simulink model "five_tank_hybrid_system"  (R2019a)
settings: Solver=FixedStepDiscrete  StartTime=0.0  StopTime=T  FixedStep=Ts  RelTol=1e-3
InitFcn:
  | load_parameters
values from neighbouring files (symbols this model uses):
  A1u = 0.0573+0.00286    (= 0.06016)    [load_parameters.m]
  A2u = 0.0573+0.00286    (= 0.06016)    [load_parameters.m]
  A3u = 0.0346+0.0017    (= 0.0363)    [load_parameters.m]
  A4u = 0.0346+0.0017    (= 0.0363)    [load_parameters.m]
  A5u = 0.0707+0.00353    (= 0.07423)    [load_parameters.m]
  Ap1u = 3.167e-5+6.33e-6    (= 3.8e-05)    [load_parameters.m]
  Ap2u = 3.167e-5+6.33e-6    (= 3.8e-05)    [load_parameters.m]
  Ap3u = 3.167e-5+6.33e-6    (= 3.8e-05)    [load_parameters.m]
  Ap4u = 3.167e-5+6.33e-6    (= 3.8e-05)    [load_parameters.m]
  Ap5u = 3.167e-5+6.33e-6    (= 3.8e-05)    [load_parameters.m]
  Av1u = 3.167e-5+6.33e-6    (= 3.8e-05)    [load_parameters.m]
  Av2u = 3.167e-5+6.33e-6    (= 3.8e-05)    [load_parameters.m]
  Av3u = 3.167e-5+6.33e-6    (= 3.8e-05)    [load_parameters.m]
  Av4u = 3.167e-5+6.33e-6    (= 3.8e-05)    [load_parameters.m]
  cp1u = 0.68-0.0675    (= 0.6125)    [load_parameters.m]
  cp2u = 0.68-0.0675    (= 0.6125)    [load_parameters.m]
  cp3u = 0.4-0.038    (= 0.362)    [load_parameters.m]
  cp4u = 0.4-0.038    (= 0.362)    [load_parameters.m]
  cp5u = 0.7-0.068    (= 0.632)    [load_parameters.m]
  cv1u = 0.62-0.0615    (= 0.5585)    [load_parameters.m]
  cv2u = 0.62-0.0615    (= 0.5585)    [load_parameters.m]
  cv3u = 0.37-0.0365    (= 0.3335)    [load_parameters.m]
  cv4u = 0.37-0.0365    (= 0.3335)    [load_parameters.m]
  g = 9.81    [load_parameters.m]
  rho1 = 0.005    [load_parameters.m]
  rho2 = 0.005    [load_parameters.m]
  rho3 = 0.005    [load_parameters.m]
  rho4 = 0.005    [load_parameters.m]
  rho5 = 0.0063    [load_parameters.m]
  Ts = 0.01    [load_parameters.m]
  v = 0.02    [load_parameters.m]
  x1_0 = 0.3    [load_parameters.m]
  X1max = 0.4    [load_parameters.m]
  X1min = 0.1    [load_parameters.m]
  X1overflow = 0.405    [load_parameters.m]
  x2_0 = 0.12    [load_parameters.m]
  X2max = 0.4    [load_parameters.m]
  X2min = 0.1    [load_parameters.m]
  X2overflow = 0.405    [load_parameters.m]
  x3_0 = 0.15    [load_parameters.m]
  X3max = 0.35    [load_parameters.m]
  X3min = 0.1    [load_parameters.m]
  X3overflow = 0.355    [load_parameters.m]
  x4_0 = 0.3    [load_parameters.m]
  X4max = 0.35    [load_parameters.m]
  X4min = 0.1    [load_parameters.m]
  X4overflow = 0.355    [load_parameters.m]
  x5_0 = 0.09    [load_parameters.m]
  X5max = 0.2    [load_parameters.m]
  X5min = 0.05    [load_parameters.m]
  X5overflow = 0.205    [load_parameters.m]
  xi = 0.02    [load_parameters.m]
undefined symbols (not defined in the file or in its folder): dfilt, DiscIntNeverNeededParam
libraries: dsparch4 x5
(part 2 of 2)

== stateflow chart five_tank_hybrid_system/A9_Valve1/Chart ==
  state Stuck_Open
    entry: q=4;
  state Close
    entry: q=1;
  state Open
    entry: q=2;
  state Stuck_Close
    entry: q=3;
  Close -> Stuck_Open [order 2] : [phi10==1]
  Open -> Stuck_Open [order 2] : [phi10==1]
  (default) -> Close
  Close -> Open [order 1] : [x3<=X3min]
  Open -> Close [order 1] : [x3>=X3max]
  Close -> Stuck_Close [order 3] : [phi9==1]
  Open -> Stuck_Close [order 3] : [phi9==1]
  data: x3 input; phi9 input; phi10 input; X3min parameter; X3max parameter; q output

== matlab function five_tank_hybrid_system/A9_Valve1/MATLAB Function ==
  data: cv input; z output; Av input; in1 input; g input
function z = fm(cv,Av,in1,g)

z = cv*Av*sqrt(2*g*in1);

== stateflow chart five_tank_hybrid_system/A10_Valve2/Chart ==
  state Stuck_Open
    entry: q=4;
  state Close
    entry: q=1;
  state Open
    entry: q=2;
  state Stuck_Close
    entry: q=3;
  Close -> Stuck_Open [order 2] : [phi12==1]
  Open -> Stuck_Open [order 2] : [phi12==1]
  (default) -> Close
  Close -> Open [order 1] : [x4<=X4min]
  Open -> Close [order 1] : [x4>=X4max]
  Close -> Stuck_Close [order 3] : [phi11==1]
  Open -> Stuck_Close [order 3] : [phi11==1]
  data: x4 input; X4max parameter; X4min parameter; phi11 input; phi12 input; q output

== matlab function five_tank_hybrid_system/A10_Valve2/MATLAB Function ==
  data: cv input; z output; Av input; in1 input; g input
function z = fm(cv,Av,in1,g)

z = cv*Av*sqrt(2*g*in1);

== stateflow chart five_tank_hybrid_system/Scenarios/Healhy Scenario/Healthy ==
  state Healthy
    entry: phi1=0;
    entry: phi2=0;
    entry: phi3=0;
    entry: phi4=0;
    entry: phi5=0;
    entry: phi6=0;
    entry: phi7=0;
    entry: phi8=0;
    entry: phi9=0;
    entry: phi10=0;
    entry: phi11=0;
    entry: phi12=0;
    entry: phi13=0;
    entry: phi14=0;
    entry: phi15=0;
    entry: phi16=0;
  (default) -> Healthy
  data: phi1 output; phi2 output; phi3 output; phi4 output; phi5 output; phi6 output; phi7 output; phi8 output; phi9 output; phi10 output; phi11 output; phi12 output; phi13 output; phi14 output; phi15 output; phi16 output

== stateflow chart five_tank_hybrid_system/Scenarios/Leak Tank 1/Leak Tank 1 ==
  state Healthy
    entry: phi1=0;
    entry: phi2=0;
    entry: phi3=0;
    entry: phi4=0;
    entry: phi5=0;
    entry: phi6=0;
    entry: phi7=0;
    entry: phi8=0;
    entry: phi9=0;
    entry: phi10=0;
    entry: phi11=0;
    entry: phi12=0;
    entry: phi13=0;
    entry: phi14=0;
    entry: phi15=0;
    entry: phi16=0;
  state Fault
    entry: phi1=1;
    entry: phi2=0;
    entry: phi3=0;
    entry: phi4=0;
    entry: phi5=0;
    entry: phi6=0;
    entry: phi7=0;
    entry: phi8=0;
    entry: phi9=0;
    entry: phi10=0;
    entry: phi11=0;
    entry: phi12=0;
    entry: phi13=0;
    entry: phi14=0;
    entry: phi15=0;
    entry: phi16=0;
  (default) -> Healthy
  Healthy -> Fault : [t>Tf]
  data: phi1 output; phi2 output; phi3 output; phi4 output; phi5 output; phi6 output; phi7 output; phi8 output; phi9 output; phi10 output; phi11 output; phi12 output; phi13 output; phi14 output; phi15 output; phi16 output; Tf input

== stateflow chart five_tank_hybrid_system/Scenarios/Leak Tank 2/Leak Tank 2 ==
  state Healthy
    entry: phi1=0;
    entry: phi2=0;
    entry: phi3=0;
    entry: phi4=0;
    entry: phi5=0;
    entry: phi6=0;
    entry: phi7=0;
    entry: phi8=0;
    entry: phi9=0;
    entry: phi10=0;
    entry: phi11=0;
    entry: phi12=0;
    entry: phi13=0;
    entry: phi14=0;
    entry: phi15=0;
    entry: phi16=0;
  state Fault
    entry: phi1=0;
    entry: phi2=1;
    entry: phi3=0;
    entry: phi4=0;
    entry: phi5=0;
    entry: phi6=0;
    entry: phi7=0;
    entry: phi8=0;
    entry: phi9=0;
    entry: phi10=0;
    entry: phi11=0;
    entry: phi12=0;
    entry: phi13=0;
    entry: phi14=0;
    entry: phi15=0;
    entry: phi16=0;
  (default) -> Healthy
  Healthy -> Fault : [t>Tf]
  data: phi1 output; phi2 output; phi3 output; phi4 output; phi5 output; phi6 output; phi7 output; phi8 output; phi9 output; phi10 output; phi11 output; phi12 output; phi13 output; phi14 output; phi15 output; phi16 output; Tf input

== stateflow chart five_tank_hybrid_system/Scenarios/Leak Tank 3/Leak Tank 2 ==
  state Healthy
    entry: phi1=0;
    entry: phi2=0;
    entry: phi3=0;
    entry: phi4=0;
    entry: phi5=0;
    entry: phi6=0;
    entry: phi7=0;
    entry: phi8=0;
    entry: phi9=0;
    entry: phi10=0;
    entry: phi11=0;
    entry: phi12=0;
    entry: phi13=0;
    entry: phi14=0;
    entry: phi15=0;
    entry: phi16=0;
  state Fault
    entry: phi1=0;
    entry: phi2=0;
    entry: phi3=1;
    entry: phi4=0;
    entry: phi5=0;
    entry: phi6=0;
    entry: phi7=0;
    entry: phi8=0;
    entry: phi9=0;
    entry: phi10=0;
    entry: phi11=0;
    entry: phi12=0;
    entry: phi13=0;
    entry: phi14=0;
    entry: phi15=0;
    entry: phi16=0;
  (default) -> Healthy
  Healthy -> Fault : [t>Tf]
  data: phi1 output; phi2 output; phi3 output; phi4 output; phi5 output; phi6 output; phi7 output; phi8 output; phi9 output; phi10 output; phi11 output; phi12 output; phi13 output; phi14 output; phi15 output; phi16 output; Tf input

== stateflow chart five_tank_hybrid_system/Scenarios/Leak Tank 4/Leak Tank 4 ==
  state Healthy
    entry: phi1=0;
    entry: phi2=0;
    entry: phi3=0;
    entry: phi4=0;
    entry: phi5=0;
    entry: phi6=0;
    entry: phi7=0;
    entry: phi8=0;
    entry: phi9=0;
    entry: phi10=0;
    entry: phi11=0;
    entry: phi12=0;
    entry: phi13=0;
    entry: phi14=0;
    entry: phi15=0;
    entry: phi16=0;
  state Fault
    entry: phi1=0;
    entry: phi2=0;
    entry: phi3=0;
    entry: phi4=1;
    entry: phi5=0;
    entry: phi6=0;
    entry: phi7=0;
    entry: phi8=0;
    entry: phi9=0;
    entry: phi10=0;
    entry: phi11=0;
    entry: phi12=0;
    entry: phi13=0;
    entry: phi14=0;
    entry: phi15=0;
    entry: phi16=0;
  (default) -> Healthy
  Healthy -> Fault : [t>Tf]
  data: phi1 output; phi2 output; phi3 output; phi4 output; phi5 output; phi6 output; phi7 output; phi8 output; phi9 output; phi10 output; phi11 output; phi12 output; phi13 output; phi14 output; phi15 output; phi16 output; Tf input

== stateflow chart five_tank_hybrid_system/Scenarios/Leak Tank 5/Leak Tank 5 ==
  state Healthy
    entry: phi1=0;
    entry: phi2=0;
    entry: phi3=0;
    entry: phi4=0;
    entry: phi5=0;
    entry: phi6=0;
    entry: phi7=0;
    entry: phi8=0;
    entry: phi9=0;
    entry: phi10=0;
    entry: phi11=0;
    entry: phi12=0;
    entry: phi13=0;
    entry: phi14=0;
    entry: phi15=0;
    entry: phi16=0;
  state Fault
    entry: phi1=0;
    entry: phi2=0;
    entry: phi3=0;
    entry: phi4=0;
    entry: phi5=1;
    entry: phi6=0;
    entry: phi7=0;
    entry: phi8=0;
    entry: phi9=0;
    entry: phi10=0;
    entry: phi11=0;
    entry: phi12=0;
    entry: phi13=0;
    entry: phi14=0;
    entry: phi15=0;
    entry: phi16=0;
  (default) -> Healthy
  Healthy -> Fault : [t>Tf]
  data: phi1 output; phi2 output; phi3 output; phi4 output; phi5 output; phi6 output; phi7 output; phi8 output; phi9 output; phi10 output; phi11 output; phi12 output; phi13 output; phi14 output; phi15 output; phi16 output; Tf input

== stateflow chart five_tank_hybrid_system/Scenarios/Pump 1 Fail/Pump 1 Fail ==
  state Healthy
    entry: phi1=0;
    entry: phi2=0;
    entry: phi3=0;
    entry: phi4=0;
    entry: phi5=0;
    entry: phi6=0;
    entry: phi7=0;
    entry: phi8=0;
    entry: phi9=0;
    entry: phi10=0;
    entry: phi11=0;
    entry: phi12=0;
    entry: phi13=0;
    entry: phi14=0;
    entry: phi15=0;
    entry: phi16=0;
  state Fault
    entry: phi1=0;
    entry: phi2=0;
    entry: phi3=0;
    entry: phi4=0;
    entry: phi5=0;
    entry: phi6=1;
    entry: phi7=0;
    entry: phi8=0;
    entry: phi9=0;
    entry: phi10=0;
    entry: phi11=0;
    entry: phi12=0;
    entry: phi13=0;
    entry: phi14=0;
    entry: phi15=0;
    entry: phi16=0;
  (default) -> Healthy
  Healthy -> Fault : [t>Tf]
  data: phi1 output; phi2 output; phi3 output; phi4 output; phi5 output; phi6 output; phi7 output; phi8 output; phi9 output; phi10 output; phi11 output; phi12 output; phi13 output; phi14 output; phi15 output; phi16 output; Tf input

== stateflow chart five_tank_hybrid_system/Scenarios/Pump 2 Fail/Pump 2 Fail ==
  state Healthy
    entry: phi1=0;
    entry: phi2=0;
    entry: phi3=0;
    entry: phi4=0;
    entry: phi5=0;
    entry: phi6=0;
    entry: phi7=0;
    entry: phi8=0;
    entry: phi9=0;
    entry: phi10=0;
    entry: phi11=0;
    entry: phi12=0;
    entry: phi13=0;
    entry: phi14=0;
    entry: phi15=0;
    entry: phi16=0;
  state Fault
    entry: phi1=0;
    entry: phi2=0;
    entry: phi3=0;
    entry: phi4=0;
    entry: phi5=0;
    entry: phi6=0;
    entry: phi7=1;
    entry: phi8=0;
    entry: phi9=0;
    entry: phi10=0;
    entry: phi11=0;
    entry: phi12=0;
    entry: phi13=0;
    entry: phi14=0;
    entry: phi15=0;
    entry: phi16=0;
  (default) -> Healthy
  Healthy -> Fault : [t>Tf]
  data: phi1 output; phi2 output; phi3 output; phi4 output; phi5 output; phi6 output; phi7 output; phi8 output; phi9 output; phi10 output; phi11 output; phi12 output; phi13 output; phi14 output; phi15 output; phi16 output; Tf input

== stateflow chart five_tank_hybrid_system/Scenarios/Pump 3 Fail/Pump 3 Fail ==
  state Healthy
    entry: phi1=0;
    entry: phi2=0;
    entry: phi3=0;
    entry: phi4=0;
    entry: phi5=0;
    entry: phi6=0;
    entry: phi7=0;
    entry: phi8=0;
    entry: phi9=0;
    entry: phi10=0;
    entry: phi11=0;
    entry: phi12=0;
    entry: phi13=0;
    entry: phi14=0;
    entry: phi15=0;
    entry: phi16=0;
  state Fault
    entry: phi1=0;
    entry: phi2=0;
    entry: phi3=0;
    entry: phi4=0;
    entry: phi5=0;
    entry: phi6=0;
    entry: phi7=0;
    entry: phi8=1;
    entry: phi9=0;
    entry: phi10=0;
    entry: phi11=0;
    entry: phi12=0;
    entry: phi13=0;
    entry: phi14=0;
    entry: phi15=0;
    entry: phi16=0;
  (default) -> Healthy
  Healthy -> Fault : [t>Tf]
  data: phi1 output; phi2 output; phi3 output; phi4 output; phi5 output; phi6 output; phi7 output; phi8 output; phi9 output; phi10 output; phi11 output; phi12 output; phi13 output; phi14 output; phi15 output; phi16 output; Tf input

== stateflow chart five_tank_hybrid_system/Scenarios/Stuck Close Valve 1/Stuck Close ==
  state Healthy
    entry: phi1=0;
    entry: phi2=0;
    entry: phi3=0;
    entry: phi4=0;
    entry: phi5=0;
    entry: phi6=0;
    entry: phi7=0;
    entry: phi8=0;
    entry: phi9=0;
    entry: phi10=0;
    entry: phi11=0;
    entry: phi12=0;
    entry: phi13=0;
    entry: phi14=0;
    entry: phi15=0;
    entry: phi16=0;
  state Fault
    entry: phi1=0;
    entry: phi2=0;
    entry: phi3=0;
    entry: phi4=0;
    entry: phi5=0;
    entry: phi6=0;
    entry: phi7=0;
    entry: phi8=0;
    entry: phi9=1;
    entry: phi10=0;
    entry: phi11=0;
    entry: phi12=0;
    entry: phi13=0;
    entry: phi14=0;
    entry: phi15=0;
    entry: phi16=0;
  (default) -> Healthy
  Healthy -> Fault : [t>Tf]
  data: phi1 output; phi2 output; phi3 output; phi4 output; phi5 output; phi6 output; phi7 output; phi8 output; phi9 output; phi10 output; phi11 output; phi12 output; phi13 output; phi14 output; phi15 output; phi16 output; Tf input

== stateflow chart five_tank_hybrid_system/Scenarios/Stuck Open Valve 1/Stuck Open ==
  state Healthy
    entry: phi1=0;
    entry: phi2=0;
    entry: phi3=0;
    entry: phi4=0;
    entry: phi5=0;
    entry: phi6=0;
    entry: phi7=0;
    entry: phi8=0;
    entry: phi9=0;
    entry: phi10=0;
    entry: phi11=0;
    entry: phi12=0;
    entry: phi13=0;
    entry: phi14=0;
    entry: phi15=0;
    entry: phi16=0;
  state Fault
    entry: phi1=0;
    entry: phi2=0;
    entry: phi3=0;
    entry: phi4=0;
    entry: phi5=0;
    entry: phi6=0;
    entry: phi7=0;
    entry: phi8=0;
    entry: phi9=0;
    entry: phi10=1;
    entry: phi11=0;
    entry: phi12=0;
    entry: phi13=0;
    entry: phi14=0;
    entry: phi15=0;
    entry: phi16=0;
  (default) -> Healthy
  Healthy -> Fault : [t>Tf]
  data: phi1 output; phi2 output; phi3 output; phi4 output; phi5 output; phi6 output; phi7 output; phi8 output; phi9 output; phi10 output; phi11 output; phi12 output; phi13 output; phi14 output; phi15 output; phi16 output; Tf input

== stateflow chart five_tank_hybrid_system/Scenarios/Stuck Close Valve 2/Stuck Close ==
  state Healthy
    entry: phi1=0;
    entry: phi2=0;
    entry: phi3=0;
    entry: phi4=0;
    entry: phi5=0;
    entry: phi6=0;
    entry: phi7=0;
    entry: phi8=0;
    entry: phi9=0;
    entry: phi10=0;
    entry: phi11=0;
    entry: phi12=0;
    entry: phi13=0;
    entry: phi14=0;
    entry: phi15=0;
    entry: phi16=0;
  state Fault
    entry: phi1=0;
    entry: phi2=0;
    entry: phi3=0;
    entry: phi4=0;
    entry: phi5=0;
    entry: phi6=0;
    entry: phi7=0;
    entry: phi8=0;
    entry: phi9=0;
    entry: phi10=0;
    entry: phi11=1;
    entry: phi12=0;
    entry: phi13=0;
    entry: phi14=0;
    entry: phi15=0;
    entry: phi16=0;
  (default) -> Healthy
  Healthy -> Fault : [t>Tf]
  data: phi1 output; phi2 output; phi3 output; phi4 output; phi5 output; phi6 output; phi7 output; phi8 output; phi9 output; phi10 output; phi11 output; phi12 output; phi13 output; phi14 output; phi15 output; phi16 output; Tf input

== stateflow chart five_tank_hybrid_system/Scenarios/Stuck Open Valve 2/Stuck Open ==
  state Healthy
    entry: phi1=0;
    entry: phi2=0;
    entry: phi3=0;
    entry: phi4=0;
    entry: phi5=0;
    entry: phi6=0;
    entry: phi7=0;
    entry: phi8=0;
    entry: phi9=0;
    entry: phi10=0;
    entry: phi11=0;
    entry: phi12=0;
    entry: phi13=0;
    entry: phi14=0;
    entry: phi15=0;
    entry: phi16=0;
  state Fault
    entry: phi1=0;
    entry: phi2=0;
    entry: phi3=0;
    entry: phi4=0;
    entry: phi5=0;
    entry: phi6=0;
    entry: phi7=0;
    entry: phi8=0;
    entry: phi9=0;
    entry: phi10=0;
    entry: phi11=0;
    entry: phi12=1;
    entry: phi13=0;
    entry: phi14=0;
    entry: phi15=0;
    entry: phi16=0;
  (default) -> Healthy
  Healthy -> Fault : [t>Tf]
  data: phi1 output; phi2 output; phi3 output; phi4 output; phi5 output; phi6 output; phi7 output; phi8 output; phi9 output; phi10 output; phi11 output; phi12 output; phi13 output; phi14 output; phi15 output; phi16 output; Tf input

== stateflow chart five_tank_hybrid_system/Scenarios/Stuck Close Valve 3/Stuck Close ==
  state Healthy
    entry: phi1=0;
    entry: phi2=0;
    entry: phi3=0;
    entry: phi4=0;
    entry: phi5=0;
    entry: phi6=0;
    entry: phi7=0;
    entry: phi8=0;
    entry: phi9=0;
    entry: phi10=0;
    entry: phi11=0;
    entry: phi12=0;
    entry: phi13=0;
    entry: phi14=0;
    entry: phi15=0;
    entry: phi16=0;
  state Fault
    entry: phi1=0;
    entry: phi2=0;
    entry: phi3=0;
    entry: phi4=0;
    entry: phi5=0;
    entry: phi6=0;
    entry: phi7=0;
    entry: phi8=0;
    entry: phi9=0;
    entry: phi10=0;
    entry: phi11=0;
    entry: phi12=0;
    entry: phi13=1;
    entry: phi14=0;
    entry: phi15=0;
    entry: phi16=0;
  (default) -> Healthy
  Healthy -> Fault : [t>Tf]
  data: phi1 output; phi2 output; phi3 output; phi4 output; phi5 output; phi6 output; phi7 output; phi8 output; phi9 output; phi10 output; phi11 output; phi12 output; phi13 output; phi14 output; phi15 output; phi16 output; Tf input

== stateflow chart five_tank_hybrid_system/Scenarios/Stuck Open Valve 3/Stuck Open ==
  state Healthy
    entry: phi1=0;
    entry: phi2=0;
    entry: phi3=0;
    entry: phi4=0;
    entry: phi5=0;
    entry: phi6=0;
    entry: phi7=0;
    entry: phi8=0;
    entry: phi9=0;
    entry: phi10=0;
    entry: phi11=0;
    entry: phi12=0;
    entry: phi13=0;
    entry: phi14=0;
    entry: phi15=0;
    entry: phi16=0;
  state Fault
    entry: phi1=0;
    entry: phi2=0;
    entry: phi3=0;
    entry: phi4=0;
    entry: phi5=0;
    entry: phi6=0;
    entry: phi7=0;
    entry: phi8=0;
    entry: phi9=0;
    entry: phi10=0;
    entry: phi11=0;
    entry: phi12=0;
    entry: phi13=0;
    entry: phi14=1;
    entry: phi15=0;
    entry: phi16=0;
  (default) -> Healthy
  Healthy -> Fault : [t>Tf]
  data: phi1 output; phi2 output; phi3 output; phi4 output; phi5 output; phi6 output; phi7 output; phi8 output; phi9 output; phi10 output; phi11 output; phi12 output; phi13 output; phi14 output; phi15 output; phi16 output; Tf input

== stateflow chart five_tank_hybrid_system/Scenarios/Stuck Close Valve 4/Stuck Close ==
  state Healthy
    entry: phi1=0;
    entry: phi2=0;
    entry: phi3=0;
    entry: phi4=0;
    entry: phi5=0;
    entry: phi6=0;
    entry: phi7=0;
    entry: phi8=0;
    entry: phi9=0;
    entry: phi10=0;
    entry: phi11=0;
    entry: phi12=0;
    entry: phi13=0;
    entry: phi14=0;
    entry: phi15=0;
    entry: phi16=0;
  state Fault
    entry: phi1=0;
    entry: phi2=0;
    entry: phi3=0;
    entry: phi4=0;
    entry: phi5=0;
    entry: phi6=0;
    entry: phi7=0;
    entry: phi8=0;
    entry: phi9=0;
    entry: phi10=0;
    entry: phi11=0;
    entry: phi12=0;
    entry: phi13=0;
    entry: phi14=0;
    entry: phi15=1;
    entry: phi16=0;
  (default) -> Healthy
  Healthy -> Fault : [t>Tf]
  data: phi1 output; phi2 output; phi3 output; phi4 output; phi5 output; phi6 output; phi7 output; phi8 output; phi9 output; phi10 output; phi11 output; phi12 output; phi13 output; phi14 output; phi15 output; phi16 output; Tf input

== stateflow chart five_tank_hybrid_system/Scenarios/Stuck Open Valve 4/Stuck Open ==
  state Healthy
    entry: phi1=0;
    entry: phi2=0;
    entry: phi3=0;
    entry: phi4=0;
    entry: phi5=0;
    entry: phi6=0;
    entry: phi7=0;
    entry: phi8=0;
    entry: phi9=0;
    entry: phi10=0;
    entry: phi11=0;
    entry: phi12=0;
    entry: phi13=0;
    entry: phi14=0;
    entry: phi15=0;
    entry: phi16=0;
  state Fault
    entry: phi1=0;
    entry: phi2=0;
    entry: phi3=0;
    entry: phi4=0;
    entry: phi5=0;
    entry: phi6=0;
    entry: phi7=0;
    entry: phi8=0;
    entry: phi9=0;
    entry: phi10=0;
    entry: phi11=0;
    entry: phi12=0;
    entry: phi13=0;
    entry: phi14=0;
    entry: phi15=0;
    entry: phi16=1;
  (default) -> Healthy
  Healthy -> Fault : [t>Tf]
  data: phi1 output; phi2 output; phi3 output; phi4 output; phi5 output; phi6 output; phi7 output; phi8 output; phi9 output; phi10 output; phi11 output; phi12 output; phi13 output; phi14 output; phi15 output; phi16 output; Tf input

== stateflow chart five_tank_hybrid_system/Scenarios/Multible/Stuck Close ==
  state Healthy
    entry: phi1=0;
    entry: phi2=0;
    entry: phi3=0;
    entry: phi4=0;
    entry: phi5=0;
    entry: phi6=0;
    entry: phi7=0;
    entry: phi8=0;
    entry: phi9=0;
    entry: phi10=0;
    entry: phi11=0;
    entry: phi12=0;
    entry: phi13=0;
    entry: phi14=0;
    entry: phi15=0;
    entry: phi16=0;
  state Fault
    entry: phi1=0;
    entry: phi2=0;
    entry: phi3=0;
    entry: phi4=0;
    entry: phi5=0;
    entry: phi6=0;
    entry: phi7=0;
    entry: phi8=1;
    entry: phi9=1;
    entry: phi10=0;
    entry: phi11=1;
    entry: phi12=0;
    entry: phi13=0;
    entry: phi14=0;
    entry: phi15=0;
    entry: phi16=0;
  (default) -> Healthy
  Healthy -> Fault : [t>Tf]
  data: phi1 output; phi2 output; phi3 output; phi4 output; phi5 output; phi6 output; phi7 output; phi8 output; phi9 output; phi10 output; phi11 output; phi12 output; phi13 output; phi14 output; phi15 output; phi16 output; Tf input

== stateflow chart five_tank_hybrid_system/Subsystem/Chart ==
  state Close
    entry: u1=0;
  state Open
    entry: u1=1;
  state Close1
    entry: u1=0;
  state Open1
    entry: u1=1;
  state Close2
    entry: u1=0;
  state Open2
    entry: u1=1;
  Close2 -> Open2 : [t>8000]
  Close1 -> Open1 : [t>780]
  Open1 -> Close2 : [t>870]
  Open -> Close1 : [t>220]
  Close -> Open : [t>170]
  (default) -> Close
  data: u1 output

== stateflow chart five_tank_hybrid_system/Subsystem1/Chart ==
  state Close
    entry: u2=0;
  state Open
    entry: u2=1;
  state Close1
    entry: u2=0;
  state Open2
    entry: u2=1;
  state Close3
    entry: u2=0;
  Open -> Close1 : [t>350]
  Close1 -> Open2 : [t>1945]
  Close -> Open : [t>300]
  Open2 -> Close3 : [t>1050]
  (default) -> Close
  data: u2 output

== matlab function five_tank_hybrid_system/A1_Tank1/MATLAB Function2 ==
  data: A input; g input; x input; f1 output
function f1 = f_leak(A,g,x)

f1 = (0.01/A)*pi*sqrt(2*g*x);
